simulink model "example_Hot_Water_Consumption_EU_tapping"  (Simulink 8.2)
settings: Solver=ode45  StartTime=0.0  StopTime=24*3600  RelTol=1e-3
libraries: carnot x3
settings Model: Creator=drhf  LastModifiedBy=drhf

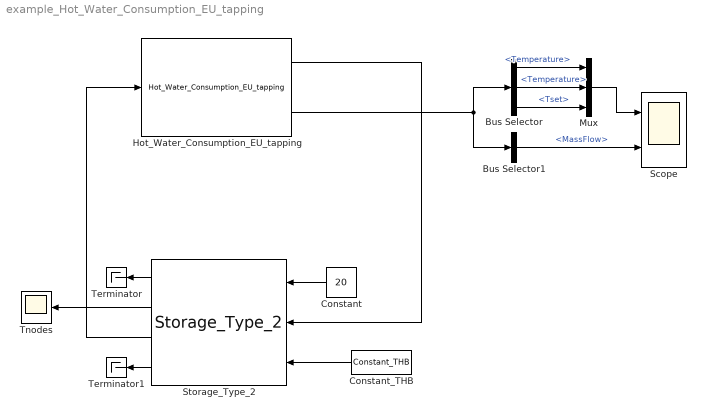
== system example_Hot_Water_Consumption_EU_tapping ==
  Bus Selector : BusSelector  OutputSignals=THBcold.Temperature,THBhot.Temperature,Tset
  Bus Selector1 : BusSelector  OutputSignals=THBhot.MassFlow
  Constant : Constant  Value=20
  Constant_THB : carnot/Source/Simple/Constant_THB  t=40  mdot=0*100/3600  p=1e5  mID=No Pressure Drop  fluid=Water  mix=0  mix2=0  mix3=0  dia=0.02  hgt=0
  Hot_Water_Consumption_EU_tapping : carnot/Load/Hot_Water_Tapping/Applications/Hot_Water_Consumption_EU_tapping  eu_tap=M  T_cold_water=10
  Mux : Mux  Inputs=3
  Scope : Scope  NumInputPorts=2
      settings: YMin=5~0  YMax=55~0.12
  Storage_Type_2 : carnot/Storage/Thermal/Storage_Type_2  uloss=1  ubot=1  utop=1  cond=1  t0=60  volume=0.3  dia=0.5  pos=standing cylinder  nconnect=2  nodes=10  mpoints=10
  Terminator : Terminator
  Terminator1 : Terminator
  Tnodes : Scope
  wires:
  Storage_Type_2/3 -> Hot_Water_Consumption_EU_tapping/1
  Storage_Type_2/1 -> Terminator/1
  Storage_Type_2/4 -> Terminator1/1
  Constant_THB/1 -> Storage_Type_2/3
  Constant/1 -> Storage_Type_2/1
  Storage_Type_2/2 -> Tnodes/1
  Hot_Water_Consumption_EU_tapping/1 -> Storage_Type_2/2
  Hot_Water_Consumption_EU_tapping/2 -> Bus Selector1/1, Bus Selector/1
  Bus Selector1/1 -> Scope/2  "<MassFlow>"
  Bus Selector/2 -> Mux/2  "<Temperature>"
  Bus Selector/3 -> Mux/3  "<Tset>"
  Bus Selector/1 -> Mux/1  "<Temperature>"
  Mux/1 -> Scope/1
